simulink library "BUS"  (R2019a)
settings: Solver=VariableStepAuto  StartTime=0.0  StopTime=10.0  RelTol=1e-3
libraries: xbsIndex_r4 x2
settings Model: Creator=Ross Donnachie  LastModifiedBy=Ross Donnachie

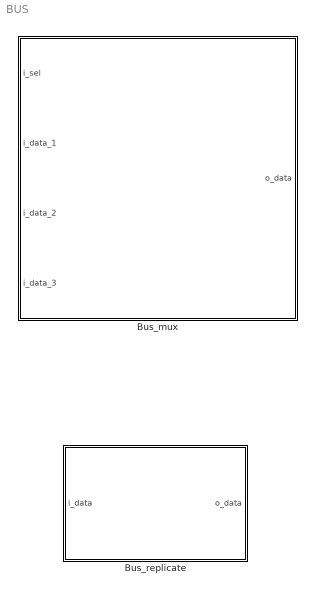
== system BUS ==
  Bus_mux : Subsystem  mask{bit_width=4, number_of_inputs=3, delay=1}
      mask prompts: bit_width "The bit-width of the ports"; number_of_inputs "The number of inputs"; delay "Latency"
      mask init:
      | Simulink.Block.eval([gcb, '/bus_mux']);
      | 
      | bus_mux_subsys2bb_knit();
      mask DialogControl DescTextVar Prompt: A generic multiplexer.
  Bus_replicate : Subsystem  mask{replication_factor=2, delay=0, misc_enabled=off}
      mask prompts: replication_factor "Replication Factor"; delay "Latency"; misc_enabled "Misc Support"
      mask DialogControl DescTextVar Prompt: Output bus formed with the input repeated in each element.

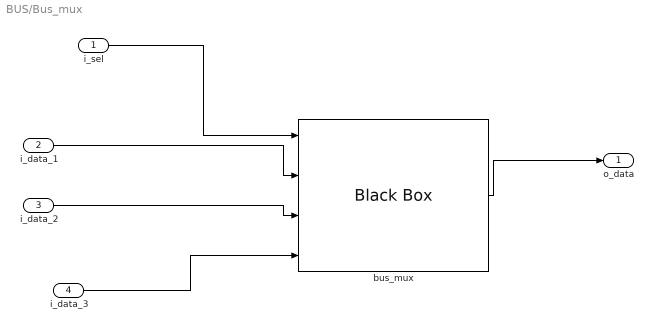
== system BUS/Bus_mux ==
  i_sel : Inport
  i_data_1 : Inport  Port=2
  i_data_2 : Inport  Port=3
  i_data_3 : Inport  Port=4
  bus_mux : xbsIndex_r4/Black Box  init_code=bus_mux_config  sim_method=ISE Simulator  verbose=off  block_type=blackbox2
  o_data : Outport
  wires:
  i_sel/1 -> bus_mux/1
  bus_mux/1 -> o_data/1
  i_data_1/1 -> bus_mux/2
  i_data_2/1 -> bus_mux/3
  i_data_3/1 -> bus_mux/4

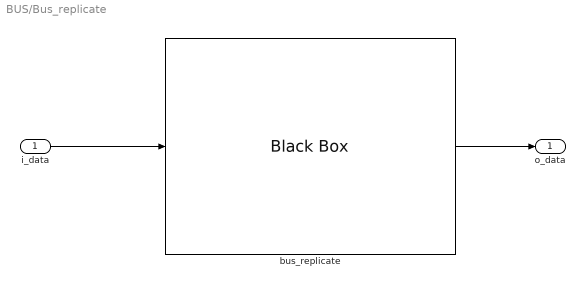
== system BUS/Bus_replicate ==
  i_data : Inport
  bus_replicate : xbsIndex_r4/Black Box  init_code=bus_replicate_config  sim_method=ISE Simulator  verbose=off  block_type=blackbox2
  o_data : Outport
  wires:
  i_data/1 -> bus_replicate/1
  bus_replicate/1 -> o_data/1
